simulink model "OMSv1_4"  (Simulink 7.0)
settings: Solver=ode4  SolverMode=SingleTasking  StartTime=0.0  StopTime=4  FixedStep=0.001  MaxStep=0.001  RelTol=1e-3  AbsTol=1e-3
PreLoadFcn:
  | setmdlp
values from neighbouring files (symbols this model uses):
  mdlparamlist = loadin.old    [setmdlp.m]
undefined symbols (not defined in the file or in its folder): alexlaw, bs_onoff, bs_scale, bsfsacrit, bsfsvcrit, cnsgain, current, fs_onoff, fs_scale, fsdelaycalc, ltdrk, phasicgain, pmcgain, pmctau2, pmctau3, saccsw, sigbuilder_block, spgain, tonicgain, tvrD, tvrN
(part 1 of 10)
CloseFcn:
  | ;slview('closediagram',bdroot);
  | try
  | close(999);
  | catch
  | end
settings Model: Creator=jacobs  LastModifiedBy=jss  ExtModeAutoUpdateStatusClock=off
settings DataIOCC: LimitDataPoints=off  SaveOutput=off  SaveTime=off
settings OptimizationCC: BlockReduction=off  BooleanDataType=off
settings DebuggingCC: SaveWithParameterizedLinksMsg=none  SignalResolutionControl=TryResolveAllWithWarning  SolverPrmCheckMsg=none  MultiTaskDSMMsg=warning  MultiTaskCondExecSysMsg=none  StrictBusMsg=None
settings HardwareCC: TargetUnknown=on
settings RTWCC: IncludeERTFirstTime=on
settings GRTTargetCC: TargetFcnLib=ansi_tfl_tmw.mat  ModelReferenceCompliant=off  MatFileLogging=off

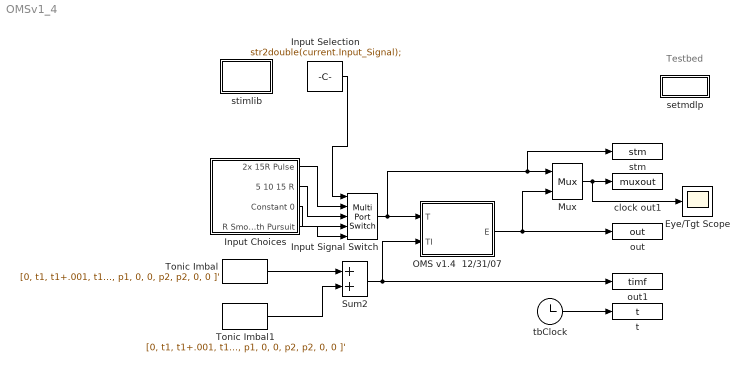
== system OMSv1_4 ==
  note: Testbed
  Eye/Tgt Scope : Scope
      settings: TickLabels=on  TimeRange=4  YMin=-2.5  YMax=17.5  DataFormat=Array
  Input Choices : Subsystem  Tag=STV Subsys  LoadFcn=sigbuilder_block('load',[437.6 199.2 550.4 400 ]);  StartFcn=sigbuilder_block('start');  StopFcn=sigbuilder_block('stop');  ClipboardFcn=sigbuilder_block('clipboard');  mask(Sigbuilder block){}
      mask help: Sigbuilder GUI
      mask init:
      | if ~strcmp(get_param(bdroot(gcbh),'SimulationStatus'),'stopped') tuvar = sigbuilder_block('maskInit'); end
      settings: CopyFcn=sigbuilder_block('copy');  DeleteFcn=sigbuilder_block('delete');  ModelCloseFcn=sigbuilder_block('modelClose');  PreSaveFcn=sigbuilder_block('preSave');  NameChangeFcn=sigbuilder_block('namechange');  OpenFcn=sigbuilder_block('open',[437.6 199.2 550.4 400 ]);  CloseFcn=sigbuilder_block('close');
      mask Display: plot(0,0,100,100,[10,10,40,40,10],[80,20,20,80,80],[40,10],[50,50], [40,27,10],[65,72,56],[40,25,25,10],[28,28,43,43]);
  Input Selection : Constant  Tag=Input_Signal  Value=str2double(current.Input_Signal);  OutDataType=sfix(16)  OutScaling=2^0
  Input Signal Switch : MultiPortSwitch  OutDataType=sfix(16)  OutScaling=2^0
  Mux : Mux  Inputs=2
  OMS v1.4  12/31/07 : Subsystem
      mask init:
      | k=0.25;loadmdlp;prolong_buffersize=5120;
      mask Display: disp('OMS v1.4\nModel')
  Sum2 : Sum  OutDataType=sfix(16)  OutScaling=2^0  SaturateOnIntegerOverflow=on  InputSameDT=on
  Tonic Imbal : FromWorkspace  VariableName=[0, t1, t1+.001, t1+d1, t1+d1+.001, t1+d1+.001+ipd, t1+d1+.001+ipd, t1+d1+.001+ipd+d2, t1+d1+.001+ipd+d2, 10000; 0, 0, p1, p1, 0, 0, p2, p2, 0, 0 ]'  SampleTime=.001  mask{@1=0, @2=0, @3=2, @4=0, @5=0, @6=3}
      mask prompts: @1 "Pulse 1 Magnitude"; @2 "Time of Pulse 1 Onset"; @3 "Pulse 1 Duration"; @4 "Interpulse Delay"; @5 "Pulse 2 Magnitude"; @6 "Pulse 2 Duration"
      mask help: Double Pulse
      mask init:
      | p1=@1; t1=@2; d1=@3; ipd=@4; p2=@5; d2=@6;
      mask Display: disp('Double\nPulse')
  Tonic Imbal1 : FromWorkspace  VariableName=[0, t1, t1+.001, t1+d1, t1+d1+.001, t1+d1+.001+ipd, t1+d1+.001+ipd, t1+d1+.001+ipd+d2, t1+d1+.001+ipd+d2, 10000; 0, 0, p1, p1, 0, 0, p2, p2, 0, 0 ]'  SampleTime=.001  mask{@1=0, @2=0, @3=3.5, @4=0, @5=0, @6=1.5}
      mask prompts: @1 "Pulse 1 Magnitude"; @2 "Time of Pulse 1 Onset"; @3 "Pulse 1 Duration"; @4 "Interpulse Delay"; @5 "Pulse 2 Magnitude"; @6 "Pulse 2 Duration"
      mask help: Double Pulse
      mask init:
      | p1=@1; t1=@2; d1=@3; ipd=@4; p2=@5; d2=@6;
      mask Display: disp('Double\nPulse')
  clock out1 : ToWorkspace  VariableName=muxout  SaveFormat=Array
      settings: MaxDataPoints=100000
  out : ToWorkspace  VariableName=out  SaveFormat=Array
      settings: MaxDataPoints=100000
  out1 : ToWorkspace  VariableName=timf  SaveFormat=Array
      settings: MaxDataPoints=100000
  setmdlp : Subsystem
      settings: OpenFcn=setmdlp
      mask Display: disp('setmdlp')
  stimlib : Subsystem
      settings: OpenFcn=stimlib
      mask Display: disp('Stimlib')
  stm : ToWorkspace  VariableName=stm  SaveFormat=Array
      settings: MaxDataPoints=100000
  t : ToWorkspace  VariableName=t  SaveFormat=Array
      mask init:
      | global t
      settings: MaxDataPoints=100000
  tbClock : Clock
      settings: Decimation=10
  wires:
  tbClock/1 -> t/1
  Input Signal Switch/1 -> OMS v1.4  12/31/07/1(T), stm/1, Mux/1
  OMS v1.4  12/31/07/1(E) -> out/1, Mux/2
  Mux/1 -> clock out1/1, Eye/Tgt Scope/1
  Tonic Imbal/1 -> Sum2/1
  Tonic Imbal1/1 -> Sum2/2
  Sum2/1 -> OMS v1.4  12/31/07/2(TI), out1/1
  Input Selection/1 -> Input Signal Switch/1
  Input Choices/1(2x 15R Pulse) -> Input Signal Switch/2
  Input Choices/2(5 10 15 R) -> Input Signal Switch/3
  Input Choices/3(Constant 0) -> Input Signal Switch/4
  Input Choices/4(R Smooth Pursuit) -> Input Signal Switch/5

== system OMSv1_4/Input Choices ==
  Demux : Demux  Tag=STV Demux
  FromWs : FromWorkspace  Tag=STV FromWs  VariableName=tuvar  SampleTime=0  SigBuilderData=DataTag0  VnvData=DataTag1
  2x 15R Pulse : Outport  Tag=STV Outport  OutDataType=sfix(16)  OutScaling=2^0
  5 10 15 R : Outport  Tag=STV Outport  Port=2
  Constant 0 : Outport  Tag=STV Outport  Port=3
  R Smooth Pursuit : Outport  Tag=STV Outport  Port=4
  wires:
  Demux/1 -> 2x 15R Pulse/1
  FromWs/1 -> Demux/1
  Demux/2 -> 5 10 15 R/1
  Demux/3 -> Constant 0/1
  Demux/4 -> R Smooth Pursuit/1

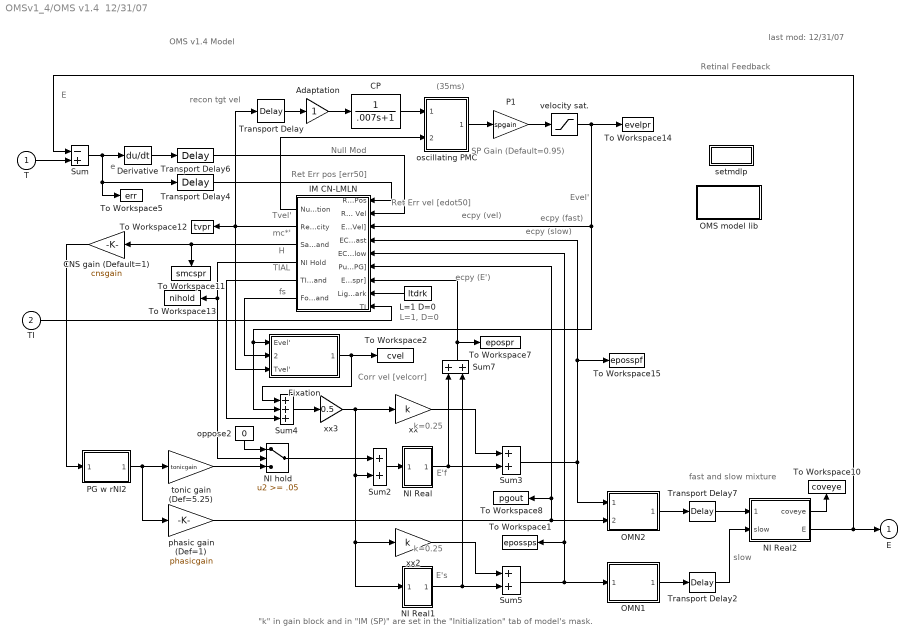
== system OMSv1_4/OMS v1.4  12/31/07 ==
  note: E'f
  note: k=0.25
  note: "k" in gain block and in "IM (SP)" are set in
      | the "Initialization" tab of model's mask.
  note: E
  note: e
  note: TIAL
  note: H
  note: mc*'
  note: Tvel'
  note: ecpy
      | (E')
  note: ecpy (vel)
  note: (35ms)
  note: Retinal Feedback
  note: recon tgt vel
  note: last mod:
      | 12/31/07
  note: Evel'
  note: OMS v1.4 Model
  note: ecpy (fast)
  note: Ret Err vel
      | [edot50]
  note: Ret Err pos [err50]
  note: SP Gain
      | (Default=0.95)
  note: L=1, D=0
  note: Corr vel
      | [velcorr]
  note: fs
  note: Null Mod
  note: E's
  note: k=0.25
  note: fast and slow
      | mixture
  note: slow
  note: ecpy (slow)
  T : Inport  OutDataType=sfix(16)  OutScaling=2^0
  TI : Inport  Port=2  OutDataType=sfix(16)  OutScaling=2^0
  Adaptation : Gain  ParameterDataType=sfix(16)  ParameterScaling=2^0  OutDataType=sfix(16)  OutScaling=2^0  SaturateOnIntegerOverflow=on
  CNS gain (Default=1) : Gain  Orientation=left  Gain=cnsgain  ParameterDataType=sfix(16)  ParameterScaling=2^0  OutDataType=sfix(16)  OutScaling=2^0  SaturateOnIntegerOverflow=on
  CP : TransferFcn  Denominator=[.007 1]
  Derivative : Derivative
      mask Display: disp('s')
  Fixation : Subsystem
      mask Display: disp('Fixation')
  IM CN-LMLN : Subsystem  Orientation=left
      mask Display: disp('INTERNAL\nMONITOR')
  L=1 D=0 : Constant  Orientation=left  Value=ltdrk  OutDataType=sfix(16)  OutScaling=2^0
  NI Real : Subsystem
      mask Display: disp('NI\nReal')
  NI Real1 : Subsystem
      mask Display: disp('NI\nReal')
  NI Real2 : Subsystem
      mask Display: disp('Plant')
  NI hold : Switch  Threshold=.05  SaturateOnIntegerOverflow=on  InputSameDT=on
  OMN1 : Subsystem
      mask Display: disp('Slow\nOMN')
  OMN2 : Subsystem
      mask Display: disp('Fast\nOMN')
  OMS model lib : Subsystem
      mask Display: disp('OMS Model\nLib')
  P1 : Gain  Gain=spgain  ParameterDataType=sfix(16)  ParameterScaling=2^0  OutDataType=sfix(16)  OutScaling=2^0  SaturateOnIntegerOverflow=on
  PG w rNI2 : Subsystem
      mask Display: disp('PG rNI 2\n(2P)')
  Sum : Sum  Inputs=-+  OutDataType=sfix(16)  OutScaling=2^0  SaturateOnIntegerOverflow=on  InputSameDT=on
  Sum2 : Sum  OutDataType=sfix(16)  OutScaling=2^0  SaturateOnIntegerOverflow=on  InputSameDT=on
  Sum3 : Sum  OutDataType=sfix(16)  OutScaling=2^0  SaturateOnIntegerOverflow=on  InputSameDT=on
  Sum4 : Sum  Inputs=+++  OutDataType=sfix(16)  OutScaling=2^0  SaturateOnIntegerOverflow=on  InputSameDT=on
  Sum5 : Sum  OutDataType=sfix(16)  OutScaling=2^0  SaturateOnIntegerOverflow=on  InputSameDT=on
  Sum7 : Sum  Orientation=up  OutDataType=sfix(16)  OutScaling=2^0  SaturateOnIntegerOverflow=on  InputSameDT=on
  To Workspace1 : ToWorkspace  VariableName=epossps  SaveFormat=Array
      settings: MaxDataPoints=10000
  To Workspace10 : ToWorkspace  VariableName=coveye  SaveFormat=Array
      settings: Orientation=up  MaxDataPoints=10000
  To Workspace11 : ToWorkspace  VariableName=smcspr  SaveFormat=Array
      settings: Orientation=down  MaxDataPoints=10000
  To Workspace12 : ToWorkspace  VariableName=tvpr  SaveFormat=Array
      settings: MaxDataPoints=10000
  To Workspace13 : ToWorkspace  VariableName=nihold  SaveFormat=Array
      settings: MaxDataPoints=10000
  To Workspace14 : ToWorkspace  VariableName=evelpr  SaveFormat=Array
      settings: MaxDataPoints=10000
  To Workspace15 : ToWorkspace  VariableName=eposspf  SaveFormat=Array
      settings: MaxDataPoints=10000
  To Workspace2 : ToWorkspace  VariableName=cvel  SaveFormat=Array
      settings: MaxDataPoints=10000
  To Workspace5 : ToWorkspace  VariableName=err  SaveFormat=Array
      settings: MaxDataPoints=10000
  To Workspace7 : ToWorkspace  VariableName=epospr  SaveFormat=Array
      settings: MaxDataPoints=10000
  To Workspace8 : ToWorkspace  VariableName=pgout  SaveFormat=Array
      settings: MaxDataPoints=10000
  Transport Delay : TransportDelay  DelayTime=0.015
      mask Display: disp('15ms')
  Transport Delay2 : TransportDelay  DelayTime=0.005
      mask Display: disp('5ms')
  Transport Delay4 : TransportDelay  DelayTime=.05
      mask Display: disp('50ms')
  Transport Delay6 : TransportDelay  DelayTime=.05
      mask Display: disp('50ms')
  Transport Delay7 : TransportDelay  DelayTime=0.005
      mask Display: disp('5ms')
  oppose2 : Constant  Orientation=down  Value=0  OutDataType=sfix(16)  OutScaling=2^0
  oscillating PMC : Subsystem
      mask Display: disp('PMC+')
  phasic gain (Def=1) : Gain  Gain=phasicgain  ParameterDataType=sfix(16)  ParameterScaling=2^0  OutDataType=sfix(16)  OutScaling=2^0  SaturateOnIntegerOverflow=on
  setmdlp : Subsystem
      settings: OpenFcn=setmdlp
      mask Display: disp('setmdlp')
  tonic gain (Def=5.25) : Gain  Gain=tonicgain  ParameterDataType=sfix(16)  ParameterScaling=2^0  OutDataType=sfix(16)  OutScaling=2^0  SaturateOnIntegerOverflow=on
  velocity sat. : Saturate  UpperLimit=90  LowerLimit=-90
  xx : Gain  Gain=k  ParameterDataType=sfix(16)  ParameterScaling=2^0  OutDataType=sfix(16)  OutScaling=2^0  SaturateOnIntegerOverflow=on
  xx2 : Gain  Gain=k  ParameterDataType=sfix(16)  ParameterScaling=2^0  OutDataType=sfix(16)  OutScaling=2^0  SaturateOnIntegerOverflow=on
  xx3 : Gain  Gain=0.5  ParameterDataType=sfix(16)  ParameterScaling=2^0  OutDataType=sfix(16)  OutScaling=2^0  SaturateOnIntegerOverflow=on
  E : Outport  OutDataType=sfix(16)  OutScaling=2^0  InitialOutput=0
  wires:
  Derivative/1 -> Transport Delay6/1
  Sum/1 -> Derivative/1, Transport Delay4/1, To Workspace5/1
  T/1 -> Sum/2
  Transport Delay4/1 -> IM CN-LMLN/1(RetErr Pos)
  Transport Delay6/1 -> IM CN-LMLN/2(RetErr Vel)
  CP/1 -> oscillating PMC/1(desired eye vel)
  oscillating PMC/1(efference copy eye vel) -> P1/1
  Transport Delay/1 -> Adaptation/1
  velocity sat./1 -> IM CN-LMLN/3(ECPY [Vel]), Sum4/2, Fixation/1(Evel'), To Workspace14/1
  P1/1 -> velocity sat./1
  Sum4/1 -> xx3/1
  PG w rNI2/1(PG [pgout]) -> tonic gain (Def=5.25)/1, phasic gain (Def=1)/1
  tonic gain (Def=5.25)/1 -> NI hold/3
  xx/1 -> Sum3/1
  NI Real/1(NIOUT [epospr]) -> Sum3/2, Sum7/1
  Sum3/1 -> OMN2/1("[eposspf]"), To Workspace15/1, IM CN-LMLN/4(ECPY Fast)
  Fixation/1(" CorrVel [velcorr]") -> To Workspace2/1, Sum4/1
  oppose2/1 -> NI hold/1
  CNS gain (Default=1)/1 -> PG w rNI2/1("[mcsprd]")
  Sum2/1 -> NI Real/1(PG + (TIAL+SP))
  OMN2/1("[psout]") -> Transport Delay7/1
  IM CN-LMLN/5(TIAL Motor Command) -> Sum4/3
  IM CN-LMLN/4(NI Hold) -> NI hold/2, To Workspace13/1
  IM CN-LMLN/3(Saccadic Motor Command) -> To Workspace11/1, CNS gain (Default=1)/1
  IM CN-LMLN/2(Reconstructed Target Velocity) -> Transport Delay/1, To Workspace12/1, Fixation/3(Tvel')
  IM CN-LMLN/1(Null Modulation) -> oscillating PMC/2(INS Gain Modulation 75)
  xx2/1 -> Sum5/1
  NI Real1/1(NIOUT [epospr]) -> Sum5/2, Sum7/2
  Transport Delay2/1 -> NI Real2/2(slow)
  Sum5/1 -> OMN1/1("[epossps] "), To Workspace1/1, IM CN-LMLN/5(ECPY Slow)
  OMN1/1("  [sout] ") -> Transport Delay2/1
  Sum7/1 -> To Workspace7/1, IM CN-LMLN/7(ECPY [epospr])
  Transport Delay7/1 -> NI Real2/1("   ")
  NI Real2/1(coveye) -> To Workspace10/1
  NI Real2/2(E) -> E/1, Sum/1
  xx3/1 -> xx/1, Sum2/2, NI Real1/1(PG + (TIAL+SP)), xx2/1
  NI hold/1 -> Sum2/1
  Adaptation/1 -> CP/1
  TI/1 -> IM CN-LMLN/9(TI)
  L=1 D=0/1 -> IM CN-LMLN/8(Light /Dark)
  phasic gain (Def=1)/1 -> OMN2/2("[pgout]"), To Workspace8/1, IM CN-LMLN/6(Pulse Gen [PG])
  IM CN-LMLN/6(Foveating Saccade Motor Command) -> Fixation/2(fs [fsmc30])

== system OMSv1_4/setmdlp ==

== system OMSv1_4/stimlib ==

== system OMSv1_4/OMS v1.4  12/31/07/Fixation ==
  note: Fixation (counter-signal)
  note: Last mod: 07/02/07
  note: Positional error is passed through a gaussian-like function whose greatest
      | response occurs between +/-0.5 deg (approx), corresponding to the sensitivity
      | of the fovea.
  note: This factor is used (with an additional gain factor) to scale the velocity error,
      | which is then subtracted from the velocity signal that is sent from the
      | common neural integrator to the ocular motor neurons.
  note: This should have the effect of reducing the high velocity error (due
      | to CN oscillation or other sources) enough to permit an extension of
      | the foveation period.
  note: Because each attempt to extend foveation caused a pulse of velocity that was
      | integrated, an error accumulated. We prevented this by adding an equivalent pulse
      | delayed until after the extended foveation (70ms).
  Evel' : Inport  OutDataType=sfix(16)  OutScaling=2^0
  fs [fsmc30] : Inport  Port=2  OutDataType=sfix(16)  OutScaling=2^0
  Tvel' : Inport  Port=3  OutDataType=sfix(16)  OutScaling=2^0
  " " : Constant  Orientation=up  Value=-1  OutDataType=sfix(16)  OutScaling=2^0
  "35 " : Subsystem  mask{prolong=35}
      mask prompts: prolong "Prolong pulse by?  (msec)"
      mask Display: disp('prolong')
  Boolify2 : Subsystem
      mask Display: disp('Boolify')
  Product : Product  Inputs=3  OutDataType=sfix(16)  OutScaling=2^0  SaturateOnIntegerOverflow=on  RndMeth=Zero  InputSameDT=on
  Product1 : Product  OutDataType=sfix(16)  OutScaling=2^0  SaturateOnIntegerOverflow=on  RndMeth=Zero  InputSameDT=on
  Product2 : Product  OutDataType=sfix(16)  OutScaling=2^0  SaturateOnIntegerOverflow=on  RndMeth=Zero  InputSameDT=on
  Sum1 : Sum  OutDataType=sfix(16)  OutScaling=2^0  SaturateOnIntegerOverflow=on  InputSameDT=on
  Sum5 : Sum  Inputs=+-  OutDataType=sfix(16)  OutScaling=2^0  SaturateOnIntegerOverflow=on  InputSameDT=on
  To Workspace1 : ToWorkspace  VariableName=cvel2  SaveFormat=Array
      settings: MaxDataPoints=10000
  To Workspace2 : ToWorkspace  VariableName=cvel1  SaveFormat=Array
      settings: MaxDataPoints=10000
  To Workspace3 : ToWorkspace  VariableName=cvel3  SaveFormat=Array
      settings: MaxDataPoints=10000
  To Workspace4 : ToWorkspace  VariableName=cvel4  SaveFormat=Array
      settings: MaxDataPoints=10000
  Transport Delay1 : TransportDelay  Orientation=down  DelayTime=0.08
      mask Display: disp('70ms')
  Transport Delay7 : TransportDelay  DelayTime=0.05
      mask Display: disp('50ms')
  Vel Sens Factor : Gain  Gain=4  ParameterDataType=sfix(16)  ParameterScaling=2^0  OutDataType=sfix(16)  OutScaling=2^0  SaturateOnIntegerOverflow=on
  WF % to be applied : Gain  ParameterDataType=sfix(16)  ParameterScaling=2^0  OutDataType=sfix(16)  OutScaling=2^0  SaturateOnIntegerOverflow=on
  on/off : Constant  Orientation=down  OutDataType=sfix(16)  OutScaling=2^0
  plantlib link6 : Subsystem
      settings: OpenFcn=fixlib
      mask Display: disp('Fix\nLib')
  velocity sensitivity N : Lookup  InputValues="[-20 -16  -12   -6  -4  4   6   12  16 20]"  Table="[0 0   0.1    0.3    1   1   0.3  0.1   0 0]"  OutDataType=sfix(16)  OutScaling=2^0  SaturateOnIntegerOverflow=on
  " CorrVel [velcorr]" : Outport  OutDataType=sfix(16)  OutScaling=2^0  InitialOutput=0
  wires:
  Sum5/1 -> WF % to be applied/1, velocity sensitivity N/1
  Transport Delay7/1 -> Sum5/1
  WF % to be applied/1 -> Product/3, To Workspace3/1
  Product1/1 -> Sum1/1, Transport Delay1/1, To Workspace2/1
  on/off/1 -> Product1/1
  Boolify2/1(Out1) -> "35 "/1(value(in))
  Vel Sens Factor/1 -> Product/2, To Workspace1/1
  velocity sensitivity N/1 -> Vel Sens Factor/1
  Product/1 -> Product1/2
  "35 "/1(value(out)) -> Product/1, To Workspace4/1
  " "/1 -> Product2/2
  Sum1/1 -> " CorrVel [velcorr]"/1
  Product2/1 -> Sum1/2
  Transport Delay1/1 -> Product2/1
  fs [fsmc30]/1 -> Boolify2/1(In1)
  Tvel'/1 -> Transport Delay7/1
  Evel'/1 -> Sum5/2

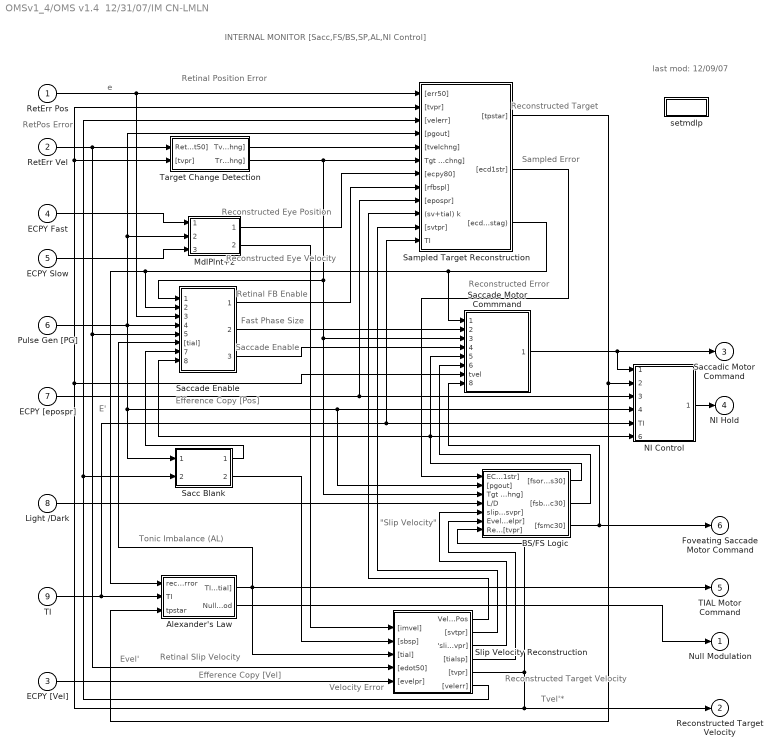
== system OMSv1_4/OMS v1.4  12/31/07/IM CN-LMLN ==
  note: INTERNAL MONITOR [Sacc,FS/BS,SP,AL,NI Control]
  note: last mod:
      | 12/09/07
  note: Reconstructed
      | Target
  note: Sampled
      | Error
  note: Reconstructed
      | Error
  note: Tonic Imbalance (AL)
  note: e
  note: Retinal Position Error
  note: RetPos
      | Error
  note: Reconstructed
      | Eye Position
  note: Reconstructed
      | Eye Velocity
  note: Retinal FB
      | Enable
  note: Saccade
      | Enable
  note: Fast Phase
      | Size
  note: Evel'
  note: Velocity Error
  note: Retinal Slip Velocity
  note: Efference Copy [Vel]
  note: Reconstructed
      | Target Velocity
  note: Tvel'*
  note: Efference Copy [Pos]
  note: E'
  note: "Slip Velocity"
  RetErr Pos : Inport  OutDataType=sfix(16)  OutScaling=2^0
  RetErr Vel : Inport  Port=2  OutDataType=sfix(16)  OutScaling=2^0
  ECPY [Vel] : Inport  Port=3  OutDataType=sfix(16)  OutScaling=2^0
  ECPY Fast : Inport  Port=4  OutDataType=sfix(16)  OutScaling=2^0
  ECPY Slow : Inport  Port=5  OutDataType=sfix(16)  OutScaling=2^0
  Pulse Gen [PG] : Inport  Port=6  OutDataType=sfix(16)  OutScaling=2^0
  ECPY [epospr] : Inport  Port=7  OutDataType=sfix(16)  OutScaling=2^0
  Light /Dark : Inport  Port=8  OutDataType=sfix(16)  OutScaling=2^0
  TI : Inport  Port=9  OutDataType=sfix(16)  OutScaling=2^0
  Alexander's Law : Subsystem
      mask Display: disp('Alexander''s\nLaw')
  BS/FS Logic : Subsystem
      mask Display: disp('Braking/Foveating\nSaccade\nLogic')
  MdlPlnt+2 : Subsystem
      mask Display: disp('Model\nPlant+')
  NI Control : Subsystem
      mask Display: disp('NI\nControl')
  Sacc Blank : Subsystem
      mask Display: disp('Saccade\n& Drift\nBlanking')
  Saccade Enable : Subsystem
      mask Display: disp('Saccade\nEnable')
  Saccade Motor Commmand : Subsystem
      mask Display: disp('Saccade\nMotor\nCommand')
  Sampled Target Reconstruction : Subsystem
      mask Display: disp('Sampled\nTarget & Error\nReconstruction')
  Slip Velocity Reconstruction : Subsystem
      mask Display: disp('Target &\nSlip Velocity\nReconstruction')
  Target Change Detection : Subsystem
      mask Display: disp('Target Change\nDetection')
  setmdlp : Subsystem
      settings: OpenFcn=setmdlp
      mask Display: disp('setmdlp')
  Null Modulation : Outport  OutDataType=sfix(16)  OutScaling=2^0  InitialOutput=0
  Reconstructed Target Velocity : Outport  Port=2  OutDataType=sfix(16)  OutScaling=2^0  InitialOutput=0
  Saccadic Motor Command : Outport  Port=3  OutDataType=sfix(16)  OutScaling=2^0  InitialOutput=0
  NI Hold : Outport  Port=4  OutDataType=sfix(16)  OutScaling=2^0  InitialOutput=0
  TIAL Motor Command : Outport  Port=5  OutDataType=sfix(16)  OutScaling=2^0  InitialOutput=0
  Foveating Saccade Motor Command : Outport  Port=6  OutDataType=sfix(16)  OutScaling=2^0  InitialOutput=0
  wires:
  NI Control/1(Hold [nihold]) -> NI Hold/1
  ECPY [epospr]/1 -> NI Control/3("[epospr]"), Sampled Target Reconstruction/9("[epospr]")
  TI/1 -> NI Control/5(TI), Sampled Target Reconstruction/12(TI), Alexander's Law/2(TI)
  Pulse Gen [PG]/1 -> Sacc Blank/1(PG [pgout]), NI Control/4(PG [pgout]), BS/FS Logic/2("[pgout]"), Saccade Enable/4("[pgout]"), Sampled Target Reconstruction/4("[pgout]"), MdlPlnt+2/2("[pgout]")
  ECPY Fast/1 -> MdlPlnt+2/1("[eposspf]")
  Alexander's Law/1(TIAL [tial]) -> Saccade Enable/6("[tial]"), Slip Velocity Reconstruction/3("[tial]"), TIAL Motor Command/1
  Saccade Motor Commmand/1("[posmc]") -> NI Control/1("[posmc]"), Saccadic Motor Command/1
  Target Change Detection/2(Trgt Chng [tchng]) -> Sampled Target Reconstruction/6(Tgt ch Det [tchng]), BS/FS Logic/3(Tgt ch Det [tchng]), Saccade Motor Commmand/3(Tgt ch Det [tchng]), Saccade Enable/1(Tgt ch Det [tchng])
  RetErr Vel/1 -> Target Change Detection/1(RetErr Vel [edot50]), Saccade Enable/5("[edot50]"), Slip Velocity Reconstruction/4("[edot50]")
  Slip Velocity Reconstruction/1(Vel->Pos) -> Sampled Target Reconstruction/10((sv+tial) k)
  Slip Velocity Reconstruction/2("[svtpr]") -> Sampled Target Reconstruction/11("[svtpr]")
  Slip Velocity Reconstruction/6("[velerr]") -> Sampled Target Reconstruction/3("[velerr]"), Sacc Blank/2(RetVelErr [velerr])
  Target Change Detection/1(Tvel Chng [tvelchng]) -> Sampled Target Reconstruction/5("[tvelchng]")
  Sampled Target Reconstruction/1("[tpstar]") -> NI Control/2(T'* [tpstar]), Alexander's Law/3(tpstar)
  RetErr Pos/1 -> Saccade Enable/3("[err50]"), Sampled Target Reconstruction/1("[err50]")
  MdlPlnt+2/1("[ecpy80]") -> Sampled Target Reconstruction/7("[ecpy80]")
  Saccade Enable/1("[rfbspl]") -> Sampled Target Reconstruction/8("[rfbspl]")
  Slip Velocity Reconstruction/5("[tvpr]") -> Reconstructed Target Velocity/1, Target Change Detection/2("[tvpr]"), Sampled Target Reconstruction/2("[tvpr]"), Saccade Motor Commmand/7(tvel), BS/FS Logic/7(Recon Tgt Vel [tvpr])
  BS/FS Logic/1("[fsorbs30]") -> NI Control/6("[fsorbs30]"), Saccade Enable/8("[fsorbs30]"), Saccade Motor Commmand/5("[fsorbs30]")
  BS/FS Logic/3("[fsmc30]") -> Foveating Saccade Motor Command/1, Saccade Motor Commmand/8(fsmc30)
  MdlPlnt+2/2("[imvel]") -> Slip Velocity Reconstruction/1("[imvel]")
  Sacc Blank/2(SP S/H [sbsp]) -> Slip Velocity Reconstruction/2("[sbsp]")
  ECPY [Vel]/1 -> Slip Velocity Reconstruction/5("[evelpr]")
  Sampled Target Reconstruction/2("[ecd1str]") -> BS/FS Logic/1(ECD1* [ecd1str])
  Light /Dark/1 -> BS/FS Logic/4(L/D)
  Slip Velocity Reconstruction/3("'slip vel\" [svpr]") -> BS/FS Logic/5(slip vel [svpr])
  Slip Velocity Reconstruction/4("[tialsp]") -> BS/FS Logic/6(Evel' [evelpr])
  Sacc Blank/1(SacBlnk [sbsac]) -> Saccade Enable/7("[sbsac]")
  Sampled Target Reconstruction/3("[ecdstrdz] (excl nystag)") -> Saccade Enable/2("[ecdstrdz]"), Alexander's Law/1(reconstructed  error), Saccade Motor Commmand/1("[ecdstrdz]")
  Saccade Enable/2(FPh Size [fphsz]) -> Saccade Motor Commmand/2("[fphsz]")
  Saccade Enable/3("[sacenab]") -> Saccade Motor Commmand/4("[sacenab]")
  BS/FS Logic/2("[fsbsmc30]") -> Saccade Motor Commmand/6("[fsbcmc30]")
  Alexander's Law/2(Null Mod) -> Null Modulation/1
  ECPY Slow/1 -> MdlPlnt+2/3("[epossps]")

== system OMSv1_4/OMS v1.4  12/31/07/NI Real ==
  note: NI Real
  PG + (TIAL+SP) : Inport  OutDataType=sfix(16)  OutScaling=2^0
  Gain : Gain  Gain=25  ParameterDataType=sfix(16)  ParameterScaling=2^0  OutDataType=sfix(16)  OutScaling=2^0  SaturateOnIntegerOverflow=on
  Gain1 : Gain  Orientation=left  ParameterDataType=sfix(16)  ParameterScaling=2^0  OutDataType=sfix(16)  OutScaling=2^0  SaturateOnIntegerOverflow=on
  Sum : Sum  OutDataType=sfix(16)  OutScaling=2^0  SaturateOnIntegerOverflow=on  InputSameDT=on
  Transfer Fcn : TransferFcn  Numerator=[1/25]  Denominator=[1 1/25]
  NIOUT [epospr] : Outport  OutDataType=sfix(16)  OutScaling=2^0  InitialOutput=0
  wires:
  PG + (TIAL+SP)/1 -> Gain/1
  Gain/1 -> Sum/2
  Sum/1 -> Transfer Fcn/1
  Gain1/1 -> Sum/1
  Transfer Fcn/1 -> Gain1/1, NIOUT [epospr]/1

== system OMSv1_4/OMS v1.4  12/31/07/NI Real1 ==
  note: NI Real
  PG + (TIAL+SP) : Inport  OutDataType=sfix(16)  OutScaling=2^0
  Gain : Gain  Gain=25  ParameterDataType=sfix(16)  ParameterScaling=2^0  OutDataType=sfix(16)  OutScaling=2^0  SaturateOnIntegerOverflow=on
  Gain1 : Gain  Orientation=left  ParameterDataType=sfix(16)  ParameterScaling=2^0  OutDataType=sfix(16)  OutScaling=2^0  SaturateOnIntegerOverflow=on
  Sum : Sum  OutDataType=sfix(16)  OutScaling=2^0  SaturateOnIntegerOverflow=on  InputSameDT=on
  Transfer Fcn : TransferFcn  Numerator=[1/25]  Denominator=[1 1/25]
  NIOUT [epospr] : Outport  OutDataType=sfix(16)  OutScaling=2^0  InitialOutput=0
  wires:
  PG + (TIAL+SP)/1 -> Gain/1
  Gain/1 -> Sum/2
  Sum/1 -> Transfer Fcn/1
  Gain1/1 -> Sum/1
  Transfer Fcn/1 -> Gain1/1, NIOUT [epospr]/1

== system OMSv1_4/OMS v1.4  12/31/07/NI Real2 ==
  note: tenot
      |  reduction
      | coefficient
  note: Plant
  note: 06/14/2007
  note: fast and slow
      | mixture
  "   " : Inport  OutDataType=sfix(16)  OutScaling=2^0
  slow : Inport  Port=2  OutDataType=sfix(16)  OutScaling=2^0
  2-PPlntSat : Subsystem
      mask Display: disp('2-P Plant\n[Sat]')
  2-pole Plant1 : ZeroPole  Zeros=[ ]  Poles=[ -1/.18 -1/.007]  Gain=[1/.18 * 1/.007]
      mask Display: disp('2-pole\nPlant')
  Sum6 : Sum  OutDataType=sfix(16)  OutScaling=2^0  SaturateOnIntegerOverflow=on  InputSameDT=on
  To Workspace15 : ToWorkspace  VariableName=psout5s  SaveFormat=Array
      settings: MaxDataPoints=10000
  xx4 : Gain  Gain=1-2*mdlparamlist(25)  ParameterDataType=sfix(16)  ParameterScaling=2^0  OutDataType=sfix(16)  OutScaling=2^0  SaturateOnIntegerOverflow=on
  coveye : Outport  OutDataType=sfix(16)  OutScaling=2^0
  E : Outport  Port=2  OutDataType=sfix(16)  OutScaling=2^0
  wires:
  Sum6/1 -> 2-pole Plant1/1, 2-PPlntSat/1(in_1), To Workspace15/1
  2-PPlntSat/1(out_1) -> coveye/1
  "   "/1 -> Sum6/1
  2-pole Plant1/1 -> E/1
  slow/1 -> xx4/1
  xx4/1 -> Sum6/2

== system OMSv1_4/OMS v1.4  12/31/07/OMN1 ==
  note: Slow OMN
  note: 06/13/2007
  "[epossps] " : Inport  OutDataType=sfix(16)  OutScaling=2^0
  "  [sout] " : Outport  OutDataType=sfix(16)  OutScaling=2^0  InitialOutput=0
  wires:
  "[epossps] "/1 -> "  [sout] "/1

== system OMSv1_4/OMS v1.4  12/31/07/OMN2 ==
  note: Fast OMN
  note: Note that the OMN properly combines the pulse with the output of the NI, by latching
      | that output to its value at the moment the pulse appears.
  note: Operation: when the pulse is active ("from PG") it activates the switch, passing the
      | upper input through to the output.  When the pulse is over, the switch changes,
      | allowing the lower input (from the NI) to pass.
  note: This block behaves like the ocular motor neurons,combining a phasic pulse (from PG)
      | with the tonic step produced by integration of the step, yielding a Pulse-Step
      | to drive the plant.
  note: 06/13/2007
  "[eposspf]" : Inport  OutDataType=sfix(16)  OutScaling=2^0
  "[pgout]" : Inport  Port=2  OutDataType=sfix(16)  OutScaling=2^0
  Abs : Abs  SaturateOnIntegerOverflow=on
  Gain _ : Gain  Gain=1.0  ParameterDataType=sfix(16)  ParameterScaling=2^0  OutDataType=sfix(16)  OutScaling=2^0  SaturateOnIntegerOverflow=on
  SampHold? : Subsystem
      mask Display: disp('H=H\nS=L')
  Sign : Subsystem
      mask Type: Sign
      mask Description: y = sign(x)
      mask Help: Sign Function:\n\t\t\ty = 1 if x > 0\n\t\t\ty = 0 if x = 0\n\t\t\ty = -1 if x < 0
      mask Display: plot(-50,-50,50,50,[-50,50],[0,0],[0,0],[-50,50],[-40,0],[-30,-30],[0,40],[30,30])
  Sum : Sum  OutDataType=sfix(16)  OutScaling=2^0  SaturateOnIntegerOverflow=on  InputSameDT=on
  Switch : Switch  Threshold=.5  SaturateOnIntegerOverflow=on  InputSameDT=on
  To Workspace15 : ToWorkspace  VariableName=psout  SaveFormat=Array
      settings: MaxDataPoints=10000
  "[psout]" : Outport  OutDataType=sfix(16)  OutScaling=2^0  InitialOutput=0
  wires:
  "[eposspf]"/1 -> SampHold?/1(Input), Switch/3
  Sign/1(out_1) -> Switch/2, SampHold?/2(S/H?)
  Gain _/1 -> Sum/1
  SampHold?/1(output) -> Sum/2
  Sum/1 -> Switch/1
  "[pgout]"/1 -> Gain _/1, Abs/1
  Switch/1 -> "[psout]"/1, To Workspace15/1
  Abs/1 -> Sign/1(in_1)

== system OMSv1_4/OMS v1.4  12/31/07/OMS model lib ==
  note: How to add your own:
  note: 1. Duplicate on of the existing library blocks above.
  note: 2. In 'Edit' menu, select 'Look under mask'. In 'Icon' tab,
      |    modify the 'disp' statement in the 'Drawing Commands' field
  note: 3. In 'Edit' menu, select "Block Properties', and select the 'Callbacks'
      | tab.  Select 'OpenFcn*' from the Callback function list on the left.
      | Change the content to the name of the library you wish to call.
  plantlib link : Subsystem
      settings: OpenFcn=plantlib
      mask Display: disp('Plant\nLib')
  plantlib link1 : Subsystem
      settings: OpenFcn=nilib
      mask Display: disp('NI\nLib')
  plantlib link2 : Subsystem
      settings: OpenFcn=imlib
      mask Display: disp('IM\nLib')
  plantlib link3 : Subsystem
      settings: OpenFcn=misclib
      mask Display: disp('Misc.\nLib')
  plantlib link4 : Subsystem
      settings: OpenFcn=cnlib
      mask Display: disp('CN\nLib')
  plantlib link5 : Subsystem
      settings: OpenFcn=lnlib
      mask Display: disp('LN\nLib')
  plantlib link6 : Subsystem
      settings: OpenFcn=fixlib
      mask Display: disp('Fix\nLib')
  plantlib link7 : Subsystem
      settings: OpenFcn=filtlib
      mask Display: disp('Filt\nLib')
  plantlib link8 : Subsystem
      settings: OpenFcn=pglib
      mask Display: disp('PG\nLib')
  stimlib : Subsystem
      settings: OpenFcn=stimlib
      mask Display: disp('Stimlib')

== system OMSv1_4/OMS v1.4  12/31/07/PG w rNI2 ==
  note: Here it is at last!  A pulse generator based on a resettable integrator (look inside the PW
      | block).  The PW function controls the switch, allowing the output of the PH function to pass
      | for the appropriate duration.
  note: The refractory latch prevents the pulse generator from responding to another stimulus until a
      | physiologically acceptable refractory period has elapsed by controlling the "Sample and Hold" block.
  note: PG with Resettable NI
  note: (Init input:0)
  "[mcsprd]" : Inport  OutDataType=sfix(16)  OutScaling=2^0
  Constant1 : Constant  Orientation=up  Value=0  OutDataType=sfix(16)  OutScaling=2^0
  PH funct : MATLABFcn  MATLABFcn=phfn2_ss
      mask Display: disp('PH\nfunction')
  PW funct : Subsystem
      mask Display: disp('PW\nfunction')
  RefLatch (Default = 50ms) : Subsystem  Orientation=left  mask{@1=50}
      mask prompts: @1 "Refractory Period (ms)"
      mask help: Refractory Latch
      mask init:
      | delay=@1;
      mask Display: disp('Refract\nLatch')
  SampHold?1 : Subsystem
      mask Display: disp('S=H\nH=L')
  Switch : Switch  Threshold=0.5  SaturateOnIntegerOverflow=on  InputSameDT=on
  loop breaker : Memory  Orientation=left
  PG [pgout] : Outport  OutDataType=sfix(16)  OutScaling=2^0  InitialOutput=0
  wires:
  Constant1/1 -> Switch/3
  Switch/1 -> loop breaker/1, PG [pgout]/1
  loop breaker/1 -> RefLatch (Default = 50ms)/1(in_1)
  SampHold?1/1(output) -> PH funct/1, PW funct/1(mcspl)
  "[mcsprd]"/1 -> SampHold?1/1(Input)
  PW funct/1(pgw) -> Switch/2
  PH funct/1 -> Switch/1
  RefLatch (Default = 50ms)/1(out_1) -> SampHold?1/2(S/H?)

== system OMSv1_4/OMS v1.4  12/31/07/oscillating PMC ==
  note: desired
      | eye accel
  note: original parameters:
      | tau3=30ms
      | tau2 = 35ms
      | fb gain = 1.1
  note: Robinson: PMC+ block
  note: motor
      | error
  note: efference
      | copy
  note: "Acceleration saturation" can be seen as a lookup table that
      | provides an acceleration for a given input velocity.  We then
      | use an integrator to convert the acceleration back to a velocity.
  note: From: Robinson DA, Gordon JL and Gordon SE
      | A model of smooth pursuit eye movements
      | Biological Cybernetics 55: 43-57,  1986
  note: By increasing feedback gain,
      | above 1.1 (about 2.2)
      | we can make this block oscillate at
      | a lower tau3 than it would otherwise.
  note: CN = 3.025
      | Norm = 1.1
  note: (Default=30ms, CN=40ms)
  note: (Default=35ms)
  note: CN
      | 825
      | 0
      | .002
      | .050
      | -925
      | .002
  note: Normal
      | 0
      | 0
      | .002
      | .050
      | 0
      | .002
  note: last mod:
      | 12/10/07
  desired eye vel : Inport  OutDataType=sfix(16)  OutScaling=2^0
  INS Gain Modulation 75 : Inport  Port=2  OutDataType=sfix(16)  OutScaling=2^0
  NI Real3 : Subsystem
      mask Display: disp('Velocity\nDeadzone')
  Product1 : Product  OutDataType=sfix(16)  OutScaling=2^0  SaturateOnIntegerOverflow=on  RndMeth=Zero  InputSameDT=on
  Sum : Sum  Inputs=-++  OutDataType=sfix(16)  OutScaling=2^0  SaturateOnIntegerOverflow=on  InputSameDT=on
  Transfer Fcn2 : TransferFcn  Numerator=[pmcgain]  Denominator=[1 0]
  Transport Delay1 : TransportDelay  DelayTime=0.025
      mask Display: disp('25ms')
  accel saturation : MATLABFcn  MATLABFcn=accsat
      mask Display: plot([-80 -4 4 80],[-120 -40 40 120], [0 0],[-120 120],[-80 80],[0 0])
  double pulse4 : FromWorkspace  VariableName=[0, t1, t1+.001, t1+d1, t1+d1+.001, t1+d1+.001+ipd, t1+d1+.001+ipd, t1+d1+.001+ipd+d2, t1+d1+.001+ipd+d2, 10000; 0, 0, p1, p1, 0, 0, p2, p2, 0, 0 ]'  SampleTime=.001  mask{@1=825, @2=0, @3=.002, @4=.050, @5=-925, @6=.002}
      mask prompts: @1 "Pulse 1 Magnitude"; @2 "Time of Pulse 1 Onset"; @3 "Pulse 1 Duration"; @4 "Interpulse Delay"; @5 "Pulse 2 Magnitude"; @6 "Pulse 2 Duration"
      mask help: Double Pulse
      mask init:
      | p1=@1; t1=@2; d1=@3; ipd=@4; p2=@5; d2=@6;
      mask Display: disp('Double\nPulse')
  tau2 : TransportDelay  DelayTime=pmctau2/1000
  tau3 : TransportDelay  Orientation=left  DelayTime=pmctau3/1000
  efference copy eye vel : Outport  OutDataType=sfix(16)  OutScaling=2^0  InitialOutput=0
  wires:
  accel saturation/1 -> tau2/1
  tau2/1 -> Transfer Fcn2/1
  Sum/1 -> accel saturation/1
  tau3/1 -> Sum/1
  desired eye vel/1 -> Sum/2, NI Real3/1(tvel)
  double pulse4/1 -> Sum/3
  Transfer Fcn2/1 -> Product1/2
  INS Gain Modulation 75/1 -> Transport Delay1/1
  Product1/1 -> tau3/1, NI Real3/2(ecpyvel)
  Transport Delay1/1 -> Product1/1
  NI Real3/1(ecpyveldz) -> efference copy eye vel/1

== system OMSv1_4/OMS v1.4  12/31/07/setmdlp ==

== system OMSv1_4/OMS v1.4  12/31/07/Fixation/35  ==
  note: init = 0
  note: init = 0
  note: 02/16/01
  note: The start of the input pulse causes the value on input 1 to be held starting when the leading
      | edge occurs, and this value remains latched until 'delay' seconds after the pulse ends (trailing edge).
  note: The two integration step delays before the S&H block's S/H (bottom) input insures
      | that the input value to be latched is available to theS&H block's top input
      | before the S&H block tries to 'hold'.
  note: Stretch the duration of an input pulse, latching it at its value at pulse onset.
  note: init Q = 0
  note: Changed from 1 to 2 delays
      | on 2/16/01 to provide insurance that
      | the signal at the S input will be available
  value(in) : Inport  OutDataType=sfix(16)  OutScaling=2^0
  " x/1000" : Constant  Orientation=up  Value=0.001  OutDataType=sfix(16)  OutScaling=2^0
  Latch1 : Subsystem  mask(Latch){@1=0}
      mask prompts: @1 "Initial State for Output "Q":"
      mask help: Latch
      mask init:
      | ini=(@1~=0);
      mask Help: Latches the S input.  When S (set) is one, the Q output  becomes one.  The output remains one until the R (reset) input becomes one, forcing the output to zero.  If both R and S are one, the latch will be in an undefined state.
      mask Display: disp('S   Q\n\nR  !Q')
  Product : Product  OutDataType=sfix(16)  OutScaling=2^0  SaturateOnIntegerOverflow=on  RndMeth=Zero  InputSameDT=on
  SampHold?2 : Subsystem
      mask Display: disp('S=L\nH=H')
  Terminator : Terminator
  Variable Transport Delay : VariableTransportDelay  MaximumDelay=10  MaximumPoints=prolong_buffersize
  leading edge detect : Subsystem
      mask Display: disp('Leading\nEdge Det')
  loop breaker2 : Memory
  loop breaker3 : Memory
  stretch : Constant  Value=prolong  OutDataType=sfix(16)  OutScaling=2^0
  trailing edge detect : Subsystem
      mask Display: disp('Trailing\nEdge Det')
  value(out) : Outport  OutDataType=sfix(16)  OutScaling=2^0  InitialOutput=0
  wires:
  " x/1000"/1 -> Product/2
  Product/1 -> Variable Transport Delay/2
  stretch/1 -> Product/1
  SampHold?2/1(output) -> value(out)/1
  trailing edge detect/1(out_1) -> Variable Transport Delay/1
  value(in)/1 -> SampHold?2/1(Input), trailing edge detect/1(in_1), leading edge detect/1(in_1)
  Latch1/1(out_1) -> loop breaker2/1
  loop breaker2/1 -> loop breaker3/1
  loop breaker3/1 -> SampHold?2/2(S/H?)
  leading edge detect/1(out_1) -> Latch1/1(in_1)
  Variable Transport Delay/1 -> Latch1/2(in_2)
  Latch1/2(out_2) -> Terminator/1

== system OMSv1_4/OMS v1.4  12/31/07/Fixation/Boolify2 ==
  In1 : Inport  OutDataType=sfix(16)  OutScaling=2^0
  Abs2 : Abs  SaturateOnIntegerOverflow=on
  direction1 : Subsystem
      mask Type: Sign
      mask Description: y = sign(x)
      mask Help: Sign Function:\n\t\t\ty = 1 if x > 0\n\t\t\ty = 0 if x = 0\n\t\t\ty = -1 if x < 0
      mask Display: plot(-50,-50,50,50,[-50,50],[0,0],[0,0],[-50,50],[-40,0],[-30,-30],[0,40],[30,30])
  Out1 : Outport  OutDataType=sfix(16)  OutScaling=2^0  InitialOutput=0
  wires:
  Abs2/1 -> direction1/1(in_1)
  In1/1 -> Abs2/1
  direction1/1(out_1) -> Out1/1

== system OMSv1_4/OMS v1.4  12/31/07/Fixation/plantlib link6 ==

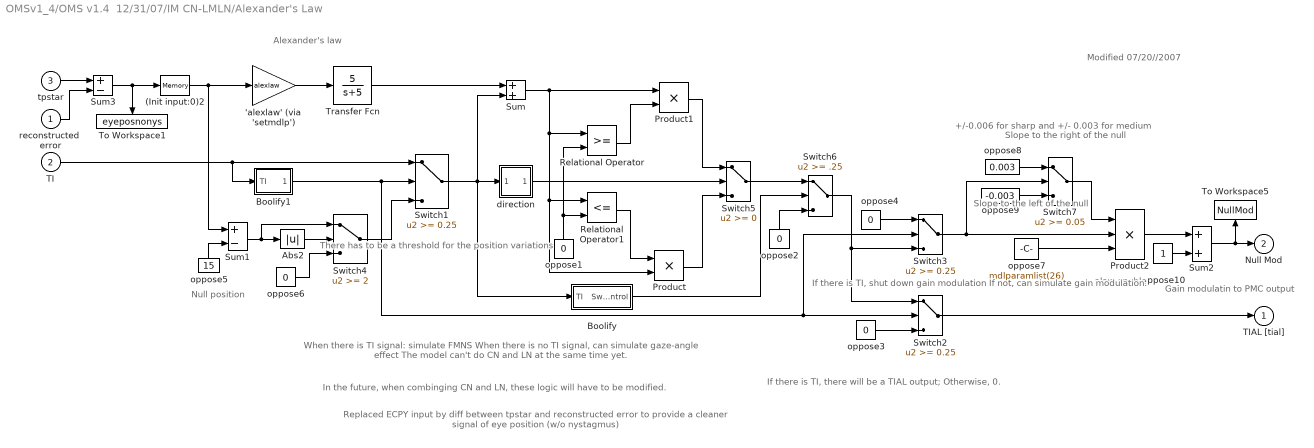
== system OMSv1_4/OMS v1.4  12/31/07/IM CN-LMLN/Alexander's Law ==
  note: Alexander's law
  note: Modified 07/20//2007
  note: Slope to the left of the null
  note: Slope to the right of the null
  note: alaw enable
  note: Gain modulatin to PMC output
  note: If there is TI, shut down gain modulation
      | If not, can simulate gain modulation.
  note: When there is TI signal: simulate FMNS
      | When there is no TI signal, can simulate gaze-angle effect
      | The model can't do CN and LN at the same time  yet.
  note: If there is TI, there will be a TIAL output;
      | Otherwise, 0.
  note: In the future, when combinging CN and LN,
      | these logic will have to be modified.
  note: There has to be
      | a threshold for the
      | position variations
  note: Null position
  note: +/-0.006 for sharp and +/- 0.003 for medium
  note: Replaced ECPY input by diff between tpstar and reconstructed error to
      | provide a cleaner signal of eye position (w/o nystagmus)
  reconstructed  error : Inport  OutDataType=sfix(16)  OutScaling=2^0
  TI : Inport  Port=2  OutDataType=sfix(16)  OutScaling=2^0
  tpstar : Inport  Port=3  OutDataType=sfix(16)  OutScaling=2^0
  'alexlaw' (via 'setmdlp') : Gain  Gain=alexlaw  ParameterDataType=sfix(16)  ParameterScaling=2^0  OutDataType=sfix(16)  OutScaling=2^0  SaturateOnIntegerOverflow=on
  (Init input:0)2 : Memory
  Abs2 : Abs  SaturateOnIntegerOverflow=on
  Boolify : Subsystem
      mask Display: disp('Boolify')
  Boolify1 : Subsystem
      mask Display: disp('Boolify')
  Product : Product  OutDataType=sfix(16)  OutScaling=2^0  SaturateOnIntegerOverflow=on  RndMeth=Zero  InputSameDT=on
  Product1 : Product  OutDataType=sfix(16)  OutScaling=2^0  SaturateOnIntegerOverflow=on  RndMeth=Zero  InputSameDT=on
  Product2 : Product  Inputs=3  OutDataType=sfix(16)  OutScaling=2^0  SaturateOnIntegerOverflow=on  RndMeth=Zero  InputSameDT=on
  Relational Operator : RelationalOperator  InputSameDT=on
  Relational Operator1 : RelationalOperator  Operator=<=  InputSameDT=on
  Sum : Sum  OutDataType=sfix(16)  OutScaling=2^0  SaturateOnIntegerOverflow=on  InputSameDT=on
  Sum1 : Sum  Inputs=+-  OutDataType=sfix(16)  OutScaling=2^0  SaturateOnIntegerOverflow=on  InputSameDT=on
  Sum2 : Sum  OutDataType=sfix(16)  OutScaling=2^0  SaturateOnIntegerOverflow=on  InputSameDT=on
  Sum3 : Sum  Inputs=+-  OutDataType=sfix(16)  OutScaling=2^0  SaturateOnIntegerOverflow=on  InputSameDT=on
  Switch1 : Switch  Threshold=0.25  SaturateOnIntegerOverflow=on  InputSameDT=on
  Switch2 : Switch  Threshold=0.25  SaturateOnIntegerOverflow=on  InputSameDT=on
  Switch3 : Switch  Threshold=0.25  SaturateOnIntegerOverflow=on  InputSameDT=on
  Switch4 : Switch  Threshold=2  SaturateOnIntegerOverflow=on  InputSameDT=on
  Switch5 : Switch  SaturateOnIntegerOverflow=on  InputSameDT=on
  Switch6 : Switch  Threshold=.25  SaturateOnIntegerOverflow=on  InputSameDT=on
  Switch7 : Switch  Threshold=0.05  SaturateOnIntegerOverflow=on  InputSameDT=on
  To Workspace1 : ToWorkspace  VariableName=eyeposnonys  SaveFormat=Array
      settings: Orientation=down  MaxDataPoints=10000
  To Workspace5 : ToWorkspace  VariableName=NullMod  SaveFormat=Array
      settings: Orientation=up  MaxDataPoints=10000
  Transfer Fcn : TransferFcn  Numerator=[5]  Denominator=[1 5]
  direction : Subsystem
      mask Type: Sign
      mask Description: y = sign(x)
      mask Help: Sign Function:\n\t\t\ty = 1 if x > 0\n\t\t\ty = 0 if x = 0\n\t\t\ty = -1 if x < 0
      mask Display: plot(-50,-50,50,50,[-50,50],[0,0],[0,0],[-50,50],[-40,0],[-30,-30],[0,40],[30,30])
  oppose1 : Constant  Orientation=up  Value=0  OutDataType=sfix(16)  OutScaling=2^0
  oppose10 : Constant  OutDataType=sfix(16)  OutScaling=2^0
  oppose2 : Constant  Orientation=up  Value=0  OutDataType=sfix(16)  OutScaling=2^0
  oppose3 : Constant  Value=0  OutDataType=sfix(16)  OutScaling=2^0
  oppose4 : Constant  Value=0  OutDataType=sfix(16)  OutScaling=2^0
  oppose5 : Constant  Orientation=up  Value=15  OutDataType=sfix(16)  OutScaling=2^0
  oppose6 : Constant  Value=0  OutDataType=sfix(16)  OutScaling=2^0
  oppose7 : Constant  Value=mdlparamlist(26)  OutDataType=sfix(16)  OutScaling=2^0
  oppose8 : Constant  Value=0.003  VectorParams1D=off  OutDataType=sfix(16)  OutScaling=2^0
  oppose9 : Constant  Value=-0.003  OutDataType=sfix(16)  OutScaling=2^0
  TIAL [tial] : Outport  OutDataType=sfix(16)  OutScaling=2^0  InitialOutput=0
  Null Mod : Outport  Port=2  OutDataType=sfix(16)  OutScaling=2^0  InitialOutput=0
  wires:
  'alexlaw' (via 'setmdlp')/1 -> Transfer Fcn/1
  Transfer Fcn/1 -> Sum/1
  Sum/1 -> Product1/1, Relational Operator1/1, Product/2, Relational Operator/1
  Relational Operator/1 -> Product1/2
  Product1/1 -> Switch5/1
  Relational Operator1/1 -> Product/1
  Product/1 -> Switch5/3
  oppose1/1 -> Relational Operator/2, Relational Operator1/2
  Switch5/1 -> Switch6/1
  oppose2/1 -> Switch6/3
  direction/1(out_1) -> Switch5/2
  Boolify/1(Switch Control) -> Switch6/2
  oppose6/1 -> Switch4/3
  Abs2/1 -> Switch4/2
  Switch4/1 -> Switch1/3
  Switch1/1 -> direction/1(in_1), Sum/2, Boolify/1(TI)
  TI/1 -> Switch1/1, Boolify1/1(TI)
  Boolify1/1(Switch Control) -> Switch1/2, Switch2/2, Switch3/2
  oppose5/1 -> Sum1/2
  Sum1/1 -> Abs2/1, Switch4/1
  oppose10/1 -> Sum2/2
  Product2/1 -> Sum2/1
  oppose8/1 -> Switch7/1
  oppose9/1 -> Switch7/3
  Switch7/1 -> Product2/1
  oppose7/1 -> Product2/3
  Sum2/1 -> Null Mod/1, To Workspace5/1
  oppose3/1 -> Switch2/3
  oppose4/1 -> Switch3/1
  Switch6/1 -> Switch3/3, Switch2/1
  Switch2/1 -> TIAL [tial]/1
  Switch3/1 -> Product2/2, Switch7/2
  (Init input:0)2/1 -> 'alexlaw' (via 'setmdlp')/1, Sum1/1
  tpstar/1 -> Sum3/1
  reconstructed  error/1 -> Sum3/2
  Sum3/1 -> (Init input:0)2/1, To Workspace1/1
